simulink model "hw11_2"  (R2018a)
settings: Solver=FixedStepAuto  StartTime=0.0  StopTime=5  FixedStep=.25  RelTol=1e-3
settings Model: Creator=mean_booty  LastModifiedBy=mean_booty
settings SolverCC: PositivePriorityOrder=on

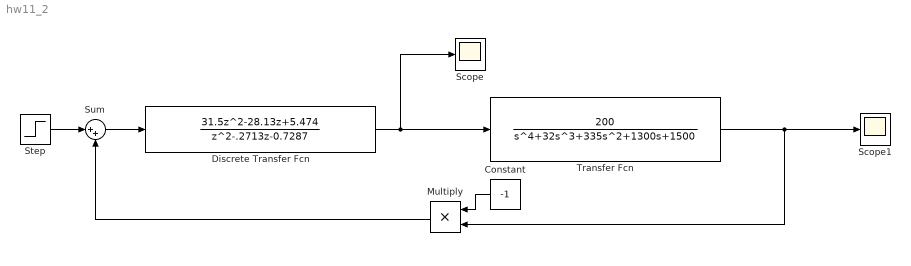
== system hw11_2 ==
  Constant : Constant  Value=-1
  Discrete Transfer Fcn : DiscreteTransferFcn  Numerator=[31.5 -28.13 5.474]  Denominator=[1 -.2713 -0.7287]
  Multiply : Product
  Scope : Scope
  Scope1 : Scope
  Step : Step  Time=0  SampleTime=0
  Sum : Sum  Inputs=|++
  Transfer Fcn : TransferFcn  Numerator=[200]  Denominator=[1 32 335 1300 1500]
  wires:
  Step/1 -> Sum/1
  Multiply/1 -> Sum/2
  Constant/1 -> Multiply/1
  Sum/1 -> Discrete Transfer Fcn/1
  Discrete Transfer Fcn/1 -> Transfer Fcn/1, Scope/1
  Transfer Fcn/1 -> Multiply/2, Scope1/1
